simulink model "LinearModel_RudderActuator3"  (R2015a)
settings: Solver=ode4  StartTime=0.0  StopTime=5  FixedStep=1e-5  RelTol=1e-3
values from neighbouring files (symbols this model uses):
  Control =     [Control.mat]
  StateControl =     [StateControl.mat]
  StateControlLinear =     [StateControlLinear.mat]
undefined symbols (not defined in the file or in its folder): EHSV_Step
settings Model: Creator=HERIC  LastModifiedBy=Pedro H
settings OptimizationCC: ExpressionDepthLimit=2147483647
settings DebuggingCC: UnderspecifiedInitializationDetection=Classic  MergeDetectMultiDrivingBlocksExec=none  SolverPrmCheckMsg=warning  StateNameClashWarn=warning

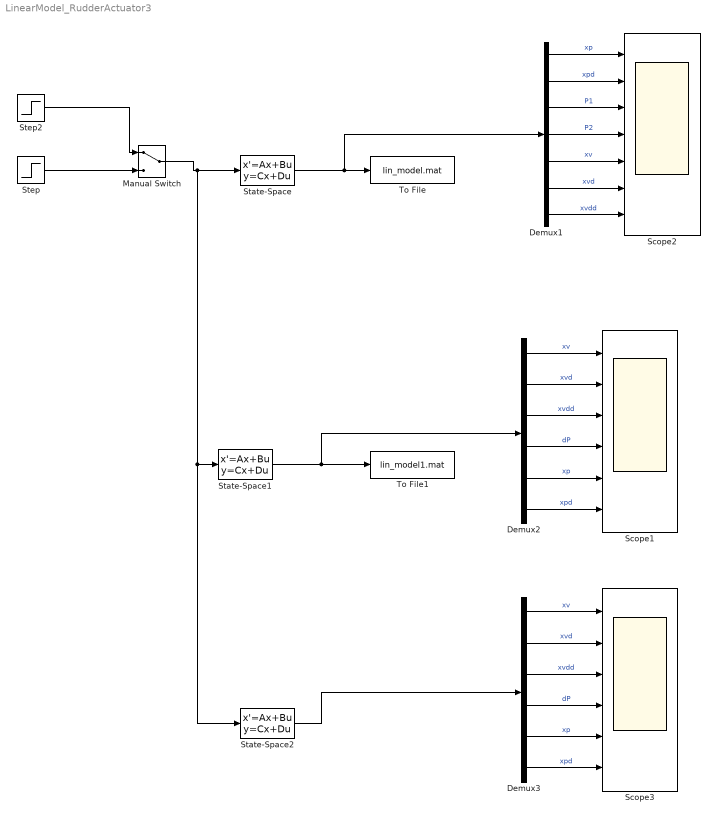
== system LinearModel_RudderActuator3 ==
  Demux1 : Demux  Outputs=7
  Demux2 : Demux  Outputs=6
  Demux3 : Demux  Outputs=6
  Manual Switch : ManualSwitch
  Scope1 : Scope  NumInputPorts=6
      settings: TimeRange=1.515675675675676  YMin=-5.9091e-26~-400000~0~-6.08696e-06~-1.15432e-20~-5e-06  YMax=0.0671053~200000~300000~3.3913e-05~0.04~5e-06
  Scope2 : Scope  NumInputPorts=7
      settings: TimeRange=1.515675675675676  YMin=-5.909099753670425e-26~-400000~0~-6.086956521739157e-06~-1.154319942386694e-20~-5e-06~-1e-09  YMax=0.06710526315789475~200000~300000~3.391304347826084e-05~0.04~5e-06~2.000000000000001e-09  SaveName=ScopeData2
  Scope3 : Scope  NumInputPorts=6
      settings: TimeRange=1.515675675675676  YMin=-5.9091e-26~-400000~0~-6.08696e-06~-1.15432e-20~-5e-06  YMax=0.0671053~200000~300000~3.3913e-05~0.04~5e-06
  State-Space : StateSpace  A=Control.A  B=Control.B  C=eye(7)  D=zeros(7,1)  X0=Control.X0
  State-Space1 : StateSpace  A=StateControl.A  B=StateControl.B  C=eye(6)  D=zeros(6,1)  X0=StateControl.X0
  State-Space2 : StateSpace  A=StateControlLinear.A  B=StateControlLinear.B  C=eye(6)  D=zeros(6,1)  X0=StateControlLinear.X0
  Step : Step  Time=EHSV_Step.time  Before=EHSV_Step.initial  After=EHSV_Step.final
  Step2 : Step  Time=0  After=10
  To File : ToFile  Filename=lin_model.mat  MatrixName=states_lin  SaveFormat=Timeseries
  To File1 : ToFile  Filename=lin_model1.mat  MatrixName=states_lin  SaveFormat=Timeseries
  wires:
  Step/1 -> Manual Switch/2
  State-Space/1 -> Demux1/1, To File/1
  Demux1/7 -> Scope2/7  "xvdd"
  Demux1/4 -> Scope2/4  "P2"
  Demux1/5 -> Scope2/5  "xv"
  Demux1/2 -> Scope2/2  "xpd"
  Demux1/1 -> Scope2/1  "xp"
  Demux1/3 -> Scope2/3  "P1"
  Manual Switch/1 -> State-Space2/1, State-Space1/1, State-Space/1
  Step2/1 -> Manual Switch/1
  Demux1/6 -> Scope2/6  "xvd"
  State-Space1/1 -> Demux2/1, To File1/1
  Demux2/5 -> Scope1/5  "xp"
  Demux2/4 -> Scope1/4  "dP"
  Demux2/3 -> Scope1/3  "xvdd"
  Demux2/1 -> Scope1/1  "xv"
  Demux2/2 -> Scope1/2  "xvd"
  Demux2/6 -> Scope1/6  "xpd"
  State-Space2/1 -> Demux3/1
  Demux3/5 -> Scope3/5  "xp"
  Demux3/4 -> Scope3/4  "dP"
  Demux3/3 -> Scope3/3  "xvdd"
  Demux3/1 -> Scope3/1  "xv"
  Demux3/2 -> Scope3/2  "xvd"
  Demux3/6 -> Scope3/6  "xpd"
